simulink model "Subsystem"  (R2020b)
settings: Solver=FixedStepAuto  StartTime=0.0  StopTime=10.0  FixedStep=0.1  RelTol=1e-3
settings Model: Creator=samar  LastModifiedBy=samar
settings DataIOCC: SaveOutput=off  SaveTime=off

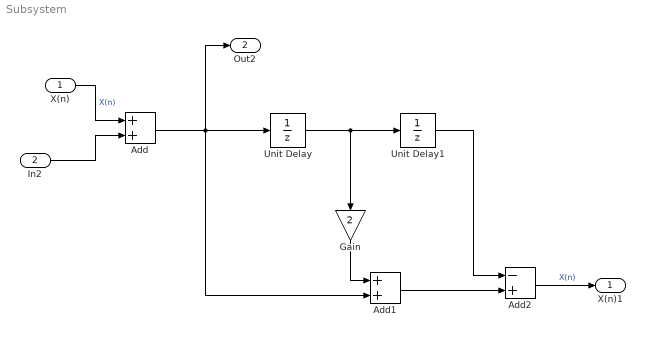
== system Subsystem ==
  X(n) : Inport  OutDataTypeStr=double  PortDimensions=1  SampleTime=[0.10000000000000001,0]
  In2 : Inport  Port=2  OutDataTypeStr=double  PortDimensions=1  SampleTime=[0.10000000000000001,0]
  Add : Sum
  Add1 : Sum
  Add2 : Sum  Inputs=-+
  Gain : Gain  Gain=2
  Unit Delay : UnitDelay  SampleTime=-1  HasFrameUpgradeWarning=on
  Unit Delay1 : UnitDelay  SampleTime=-1  HasFrameUpgradeWarning=on
  X(n)1 : Outport  OutDataTypeStr=double  PortDimensions=1  SampleTime=[0.10000000000000001,0]
  Out2 : Outport  Port=2  OutDataTypeStr=double  PortDimensions=1  SampleTime=[0.10000000000000001,0]
  wires:
  Add/1 -> Add1/2, Unit Delay/1, Out2/1
  Unit Delay/1 -> Unit Delay1/1, Gain/1
  In2/1 -> Add/2
  Gain/1 -> Add1/1
  X(n)/1 -> Add/1  "X(n)"
  Unit Delay1/1 -> Add2/1
  Add2/1 -> X(n)1/1  "X(n)"
  Add1/1 -> Add2/2
